simulink model "Gen_Sink_RS232_HFC_1P"  (Simulink 7.8)
settings: Solver=VariableStepDiscrete  StartTime=0.0  StopTime=Inf  FixedStep=Ts/4  RelTol=1e-3
PreLoadFcn:
  | clear all;
  | close all;
  | clc;
  | 
  | Ts = 1;          % clk (period)
  | 
  | Ns =  100;      % Characters to Tx and to Rx
  | minV = 0;       %  minimum data value
  | maxV = 255;       %  minimum data value
  | Tx_array = randi([minV maxV], 1, Ns, 'uint8');
  | Rx_array = randi([minV maxV], 1, Ns, 'uint8');
StartFcn:
  | clc;
  | close all;
  | 
  | %
  | %   RS232 port initialization
  | %
  | PORTNAME = 'COM56';
  | fprintf('\nOpening RS232 port %s ...... ', PORTNAME);
  | s2 = serial(PORTNAME,'BaudRate',9600,'Parity','none','DataBits',8);
  | set(s2, 'FlowControl', 'none');
  | set(s2, 'InputBufferSize', 64);
  | set(s2, 'OutputBufferSize', 1);
  | fopen(s2);
  | s1.RecordDetail = 'verbose';
  | s1.RecordName = 'uart2.txt';
  | record(s2,'on')
  | fprintf('\nRS232 port %s activated\n', PORTNAME);
  | 
  | b2o_s2 = uint8(0);
  | d2o_s2 = uint8(0);
  | b2r_s2 = uint8(0);
  | d2r_s2 = uint8(0);
  | rts_s2 = uint8(0);
  | cts_s2 = uint8(0);
StopFcn:
  | %
  | %   RS232 ports release
  | %
  | disp(' ');
  | disp('Deactivating RS232 port ......');
  | 
  | fclose(s2)
  | delete(s2)
  | clear s2
  | 
  | fprintf('RS232 port %s deactivated\n', PORTNAME);
  | 
  | if Tx_array == Rx_array
  |   disp('Data exchange without errors');
  | else
  |    Ne = sum((Tx_array - Rx_array) ~= 0);
  |    fprintf('\nData exchange with %d errors in %d data charactes\n\n', Ne, Ns);
  | end
libraries: simulink x3
settings Model: Creator=theodore  LastModifiedBy=theodore
settings DebuggingCC: SolverPrmCheckMsg=none
settings CodeAppCC: CustomSymbolStrType=$N$R$M_T

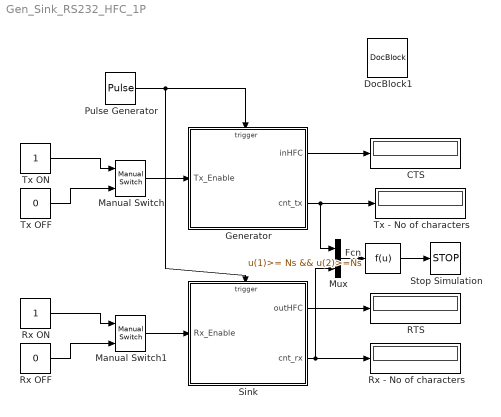
== system Gen_Sink_RS232_HFC_1P ==
  CTS : Display
  DocBlock1 : simulink/Model-Wide Utilities/DocBlock  DocumentType=Text
      content=|
      | Generator using RTS  and Sink using CTS
  Fcn : Fcn  Expr=u(1)>= Ns && u(2)>=Ns
  Generator : Stateflow chart  TreatAsAtomicUnit=on
  Manual Switch : simulink/Signal Routing/Manual Switch  sw=1  action=0  varsize=off
  Manual Switch1 : simulink/Signal Routing/Manual Switch  sw=1  action=0  varsize=off
  Mux : Mux  Inputs=2
  Pulse Generator : DiscretePulseGenerator  PulseType=Time based  Period=Ts  PulseWidth=50
  RTS : Display
  Rx - No of characters : Display
  Rx OFF : Constant  Value=0
  Rx ON : Constant
  Sink : Stateflow chart  TreatAsAtomicUnit=on
  Stop Simulation : Stop
  Tx - No of characters : Display
  Tx OFF : Constant  Value=0
  Tx ON : Constant
  wires:
  Pulse Generator/1 -> Generator/Trigger, Sink/Trigger
  Sink/2(cnt_rx) -> Rx - No of characters/1, Mux/2
  Sink/1(outHFC) -> RTS/1
  Generator/1(inHFC) -> CTS/1
  Generator/2(cnt_tx) -> Tx - No of characters/1, Mux/1
  Manual Switch/1 -> Generator/1(Tx_Enable)
  Tx ON/1 -> Manual Switch/1
  Tx OFF/1 -> Manual Switch/2
  Rx ON/1 -> Manual Switch1/1
  Rx OFF/1 -> Manual Switch1/2
  Manual Switch1/1 -> Sink/1(Rx_Enable)
  Fcn/1 -> Stop Simulation/1
  Mux/1 -> Fcn/1

== stateflow chart Sink ==
  state HFC_states [parallel]
    settings: executionOrder=1
    state HFCcon
      LBstatus_rx = Rx_Enable;
      ml.rts_s2 = LBstatus_rx;
      outHFC = LBstatus_rx;
      ml('RTS_2');
    state S1
      LBstatus_rx = Rx_Enable;
    state S2
    (default) -> HFCcon
    (junction 11) -> S1 [order 1] : [LBstatus_rx == 0]
    S1 -> (junction 12)
    S2 -> HFCcon
    HFCcon -> (junction 11)
    (junction 11) -> HFCcon [order 2]
    (junction 12) -> HFCcon [order 2]
    (junction 12) -> S2 [order 1] : [LBstatus_rx == 0]
  state Rx [parallel]
    settings: executionOrder=2
    state RxState
      en: ml('DIn_2');
      Val_rx = ml.d2r_s2;
      cnt_rx = cnt_rx + 1;
      ml.Rx_array[cnt_rx] = Val_rx;
    state IniState
    (default) -> IniState : {cnt_rx = 0;}
    (junction 10) -> IniState [order 1] : [ml.b2r_s2 == 0 ]
    (junction 10) -> RxState [order 2]
    IniState -> (junction 10) : {ml('B2R_2'); }
    RxState -> IniState
  data: outHFC output double; Val_rx local uint8; cnt_rx output double; LBstatus_rx local double =0; Rx_Enable input double
  events: CLK input RISING_EDGE_EVENT

== stateflow chart Generator ==
  state Dcalc
    en: ml('CTS_2');
    LBstatus_tx = ml.cts_s2;
    inHFC = LBstatus_tx;
  state IniState
    ml('CTS_2');
    LBstatus_tx = ml.cts_s2;
    inHFC = LBstatus_tx;
  state TxState
    en: cnt_tx = cnt_tx + 1;
    Val_tx = ml.Tx_array[cnt_tx];
    ml.d2o_s2 = Val_tx;
    ml('DOut_2');
  state Idle
  (junction 39) -> TxState [order 1] : [LBstatus_tx  ~= 0  && Tx_Enable == 1 ]
  (junction 38) -> Dcalc [order 2]
  (default) -> IniState : {cnt_tx = 0;}
  (junction 38) -> IniState [order 1] : [ml.b2o_s2 > 0 || LBstatus_tx == 0 || Tx_Enable == 0]
  TxState -> (junction 40)
  IniState -> (junction 38) : {ml('B2O_2'); }
  Dcalc -> (junction 39)
  (junction 39) -> Dcalc [order 2]
  (junction 40) -> Idle [order 1] : [cnt_tx == ml.Ns]
  (junction 40) -> IniState [order 2]
  data: inHFC output double; cnt_tx output double; Val_tx local uint8; LBstatus_tx local double =0; Tx_Enable input double
  events: CLK input RISING_EDGE_EVENT
